simulink model "zad333d_Sim"  (Simulink 7.1)
settings: Solver=ode45  StartTime=0.0  StopTime=10.0  RelTol=1e-3
settings Model: Creator=mestar  LastModifiedBy=mestar
settings DebuggingCC: SolverPrmCheckMsg=none

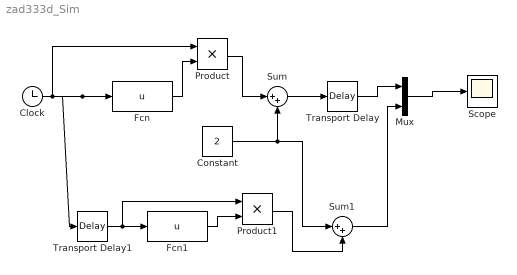
== system zad333d_Sim ==
  Clock : Clock
      settings: Decimation=10
  Constant : Constant  Value=2  OutDataType=sfix(16)  OutScaling=2^0
  Fcn : Fcn  Expr=u
  Fcn1 : Fcn  Expr=u
  Mux : Mux  Inputs=2
  Product : Product  OutDataType=sfix(16)  OutScaling=2^0  RndMeth=Zero
  Product1 : Product  OutDataType=sfix(16)  OutScaling=2^0  RndMeth=Zero
  Scope : Scope
  Sum : Sum  Inputs=|++  OutDataType=sfix(16)  OutScaling=2^0
  Sum1 : Sum  Inputs=|++  OutDataType=sfix(16)  OutScaling=2^0
  Transport Delay : TransportDelay
  Transport Delay1 : TransportDelay
  wires:
  Clock/1 -> Product/1, Fcn/1, Transport Delay1/1
  Constant/1 -> Sum/2, Sum1/1
  Fcn/1 -> Product/2
  Sum/1 -> Transport Delay/1
  Transport Delay1/1 -> Fcn1/1, Product1/1
  Transport Delay/1 -> Mux/1
  Sum1/1 -> Mux/2
  Mux/1 -> Scope/1
  Product/1 -> Sum/1
  Fcn1/1 -> Product1/2
  Product1/1 -> Sum1/2
